simulink model "LAB4"  (R2019a)
settings: Solver=VariableStepAuto  StartTime=0.0  StopTime=500.0  RelTol=1e-3
settings Model: Creator=swastik  LastModifiedBy=swastik
settings DataIOCC: ReturnWorkspaceOutputs=off
settings DebuggingCC: ArithmeticOperatorsInVariantConditions=warning

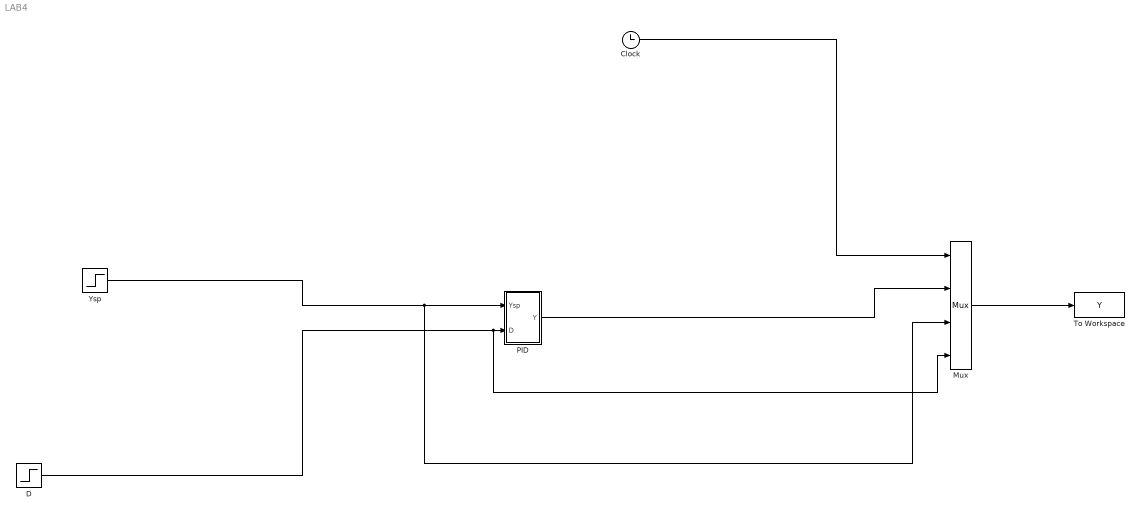
== system LAB4 ==
  Clock : Clock
  D : Step  Time=0  SampleTime=0
  Mux : Mux
  "PID " : Subsystem  mask{Kc=0.546, Ti=1e10, Td=1e-10}
      mask prompts: Kc "Controller Gain"; Ti "Integral Time"; Td "Derivative Time"
  To Workspace : ToWorkspace  VariableName=Y  SampleTime=-1
  Ysp : Step  Time=0  After=0  SampleTime=0
  wires:
  Clock/1 -> Mux/1
  Mux/1 -> To Workspace/1
  "PID "/1(Y) -> Mux/2
  Ysp/1 -> "PID "/1(Ysp), Mux/3
  D/1 -> Mux/4, "PID "/2(D)

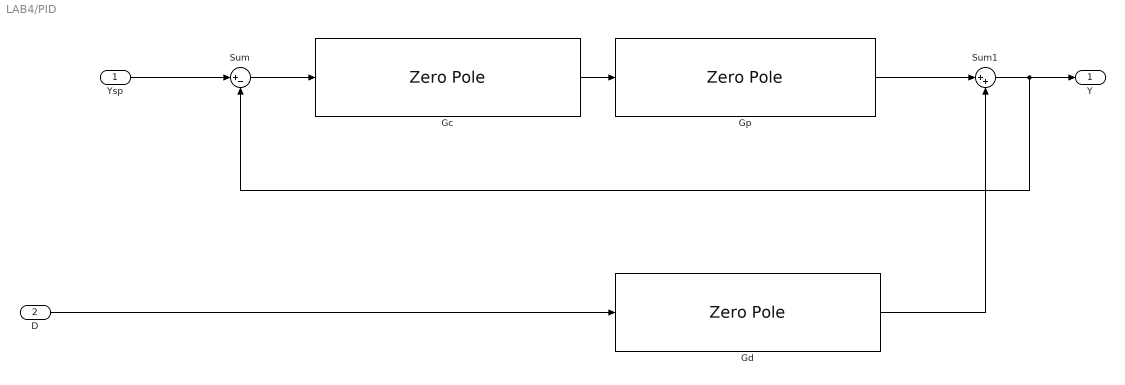
== system LAB4/PID  ==
  Ysp : Inport
  D : Inport  Port=2
  Gc : ZeroPole  Zeros=[-1/Ti -1/Td]  Poles=[0 -10/Td]  Gain=Kc/0.1
  Gd : ZeroPole  Zeros=[]  Poles=[-1/10 -1/5 -1/2 -1]  Gain=[1/100]
  Gp : ZeroPole  Zeros=[]  Poles=[-1/5 -1/2 -1 -2]  Gain=[1/2]
  Sum : Sum  Inputs=|+-
  Sum1 : Sum  Inputs=|++
  Y : Outport
  wires:
  Gc/1 -> Gp/1
  Sum1/1 -> Sum/2, Y/1
  Gd/1 -> Sum1/2
  Gp/1 -> Sum1/1
  Sum/1 -> Gc/1
  Ysp/1 -> Sum/1
  D/1 -> Gd/1
